simulink model "IndustrialMicrogrid"  (R2023a)
settings: Solver=FixedStepDiscrete  StartTime=0.0  StopTime=10  FixedStep=Ts  RelTol=1e-3
PostLoadFcn:
  | IndustrialMicrogridInputData
  | GfmGridFormingConverterInputParameters
model workspace (MAT data in the model file):
  caseNum = 2
undefined symbols (not defined in the file): base, BESS, DiscIntNeverNeededParam, grid, Grid, gridInverter, machine, microgrid, PV, PVInverter, PVTransformer, scrFactorRg, scrFactorXg, transformer, Ts
libraries: ee_lib x112, eeGeneralControl x104, nesl_utility_internal x64, simulink x56, nesl_utility x37, fl_lib x29, slpidlib x13, eeTransforms x11, eeTotalHarmonicDistorsion x8, eeRmsMeasurement x4, eeSinusoidalMeasurement x4, simulink_extras x2
(part 11 of 14)

== system IndustrialMicrogrid/Operator Room/OperatorControlRoom/MG1 Controller : Commands and Measurements/Microgrid Controller 1 : Commands and Measurements/Monitoring of system performance/Microgrid ==
  Frequency : Inport
  Voltage : Inport  Port=2
  Constant : Constant  Value=0
  Constant4 : Constant  Value=0
  Island Frequency MINMAX : Scope  NumInputPorts=4
  Island Voltage MINMAX : Scope  NumInputPorts=4
  MinMax Running Resettable : simulink/Math Operations/MinMax Running Resettable  Function=max  vinit=grid.frequency
  MinMax Running Resettable2 : simulink/Math Operations/MinMax Running Resettable  Function=max  vinit=1
  MinMax Running Resettable3 : simulink/Math Operations/MinMax Running Resettable  Function=min  vinit=1
  MinMax Running Resettable4 : simulink/Math Operations/MinMax Running Resettable  Function=min  vinit=grid.frequency
  Subsystem : Subsystem
  Subsystem3 : Subsystem
  start at 0.2 s1 : Subsystem
  start at 0.2 s3 : Subsystem
  wires:
  Subsystem/1(Out1) -> Island Frequency MINMAX/1  "Microgrid Frequency Croosed Low (59 HZ)"
  Constant/1 -> MinMax Running Resettable4/2, MinMax Running Resettable/2
  Frequency/1 -> start at 0.2 s3/1(In1)
  Subsystem3/1(Out1) -> Island Voltage MINMAX/1  "Microgrid Voltage Crossed Low (0.95 pu)"
  Subsystem/2(Out2) -> Island Frequency MINMAX/2  "Microgrid Frequency Crossed High (62 Hz)"
  Voltage/1 -> start at 0.2 s1/1(In1)
  MinMax Running Resettable2/1 -> Island Voltage MINMAX/3  "Microgrid Voltage Max (pu)"
  start at 0.2 s3/1(u) -> Subsystem/1(u), MinMax Running Resettable4/1, MinMax Running Resettable/1
  Subsystem3/2(Out2) -> Island Voltage MINMAX/2  "Microgrid Voltage Crossed High (1.1 pu)"
  start at 0.2 s1/1(u) -> MinMax Running Resettable3/1, MinMax Running Resettable2/1, Subsystem3/1(u)
  Constant4/1 -> MinMax Running Resettable3/2, MinMax Running Resettable2/2
  MinMax Running Resettable4/1 -> Island Frequency MINMAX/4  "Microgrid Frequency Min (Hz)"
  MinMax Running Resettable3/1 -> Island Voltage MINMAX/4  "Microgrid Voltage Min (pu)"
  MinMax Running Resettable/1 -> Island Frequency MINMAX/3  "Microgrid Frequency Max (Hz)"

== system IndustrialMicrogrid/Operator Room/OperatorControlRoom/MG1 Controller : Commands and Measurements/Microgrid Controller 1 : Commands and Measurements/Monitoring of system performance/Subsystem ==
  Active and Reactive Power : Inport
  In Bus Element1 : Inport  Port=2  PortName=mtieline1  Element=activepower
  In Bus Element6 : Inport  Port=2  PortName=mtieline1  Element=reactivepower
  In Bus Element2 : Inport  Port=3  PortName=mLoad3  Element=activepower
  In Bus Element3 : Inport  Port=3  PortName=mLoad3  Element=reactivepower
  Bus Selector : BusSelector  OutputSignals=signal1.Grid Active Power,signal1.BESS Active Power,signal1.Load Active Power,signal2.Grid Reactive Power,signal2.BESS Reactive Power,signal2.Load Reactive Power
  Constant4 : Constant  Value=0
  MinMax Running Resettable1 : simulink/Math Operations/MinMax Running Resettable  Function=max  vinit=0
  MinMax Running Resettable2 : simulink/Math Operations/MinMax Running Resettable  Function=max  vinit=0
  Sum : Sum  Inputs=++---
  Sum1 : Sum  Inputs=++---
  Terminator : Terminator
  Terminator1 : Terminator
  start at 2.5 s : Subsystem
  start at 2.5 s1 : Subsystem
  wires:
  start at 2.5 s1/1(u) -> MinMax Running Resettable2/1
  Constant4/1 -> MinMax Running Resettable1/2, MinMax Running Resettable2/2
  Sum/1 -> start at 2.5 s1/1(ActivePower)
  Sum1/1 -> start at 2.5 s/1(ReactivePower)
  Active and Reactive Power/1 -> Bus Selector/1
  MinMax Running Resettable2/1 -> Terminator/1  "Max Active Power Loss (kW)"
  start at 2.5 s/1(u) -> MinMax Running Resettable1/1
  MinMax Running Resettable1/1 -> Terminator1/1  "Max Active Power Loss (kW)"
  Bus Selector/1 -> Sum/1  "<Grid Active Power>"
  Bus Selector/2 -> Sum/2  "<BESS Active Power>"
  Bus Selector/3 -> Sum/3  "<Load Active Power>"
  Bus Selector/4 -> Sum1/1  "<Grid Reactive Power>"
  Bus Selector/5 -> Sum1/2  "<BESS Reactive Power>"
  Bus Selector/6 -> Sum1/3  "<Load Reactive Power>"
  In Bus Element1/1 -> Sum/4
  In Bus Element6/1 -> Sum1/4
  In Bus Element2/1 -> Sum/5
  In Bus Element3/1 -> Sum1/5

== system IndustrialMicrogrid/Operator Room/OperatorControlRoom/MG1 Controller : Commands and Measurements/Microgrid Controller 1 : Commands and Measurements/Monitoring of system performance/THD ==
  mLoad : Inport
  In2 : Inport  Port=2
  MGController : Inport  Port=3
  In4 : Inport  Port=4
  THD : Scope  NumInputPorts=4
  Total Harmonic Distortion{,1..3} (4 alike) : eeTotalHarmonicDistorsion/Total Harmonic Distortion  f=60  Ts=Ts
      settings: LibrarySourceBlock=|
      | ee_sl_lib/Measurements/Total Harmonic
      | Distortion
  wires:
  Total Harmonic Distortion1/1 -> THD/2  "Load Current THD (%)"
  Total Harmonic Distortion3/1 -> THD/4  "PCC Current THD (%)"
  Total Harmonic Distortion2/1 -> THD/3  "PCC Voltage THD (%)"
  Total Harmonic Distortion/1 -> THD/1  "Load Voltage THD (%)"
  In2/1 -> Total Harmonic Distortion1/1
  mLoad/1 -> Total Harmonic Distortion/1
  MGController/1 -> Total Harmonic Distortion2/1
  In4/1 -> Total Harmonic Distortion3/1

== system IndustrialMicrogrid/Operator Room/OperatorControlRoom/MG2 Controller : Commands and Measurements/Microgrid Controller 2 : Commands and Measurements/Measurements and visualizations 1/BESS, PV and Load Measurements ==
  Grid Active Power : Inport
  Grid Reactive Power : Inport  Port=2
  Vpv (V) : Inport  Port=3
  BESS Active Power : Inport  Port=4
  BESS Voltage : Inport  Port=5
  BESS Current : Inport  Port=6
  Load Active Power : Inport  Port=7
  Ipv (A) : Inport  Port=8
  PV Active Power : Inport  Port=9
  BESS Reactive Power : Inport  Port=10
  PV Reactive Power : Inport  Port=11
  Load Reactive Power : Inport  Port=12
  Load Current(p.u.) : Inport  Port=13
  Load Voltage (p.u.) : Inport  Port=14
  Load Voltage RMS (p.u.) : Inport  Port=15
  Diesel Active Power : Inport  Port=16
  Diesel Reactive Power : Inport  Port=17
  Active and reactive Power : Subsystem
  BESS and PV Measurements : Subsystem
  Load Active Power2 : InportShadow  Port=7
  Load Measurements : Subsystem
  Load Reactive Power1 : InportShadow  Port=12
  PV Active Power1 : InportShadow  Port=9
  PV Reactive Power1 : InportShadow  Port=11
  Active Power : Outport
  Reactive Power : Outport  Port=2
  wires:
  PV Reactive Power1/1 -> Active and reactive Power/8(PV Reactive Power)
  PV Active Power1/1 -> Active and reactive Power/4(PV Active Power)
  PV Active Power/1 -> BESS and PV Measurements/5(PV Active Power)
  Vpv (V)/1 -> BESS and PV Measurements/1(Vpv (V))
  PV Reactive Power/1 -> BESS and PV Measurements/6(PV Reactive Power)
  BESS Voltage/1 -> BESS and PV Measurements/2(Vabc)
  BESS Active Power/1 -> Active and reactive Power/2(BESS Active Power)
  BESS Current/1 -> BESS and PV Measurements/3(Iabc)
  Load Voltage RMS (p.u.)/1 -> Load Measurements/5(Load Voltage RMS (p.u.))
  Load Voltage (p.u.)/1 -> Load Measurements/4(Load Voltage (p.u.))
  Grid Active Power/1 -> Active and reactive Power/1(Grid Active Power)
  Load Active Power2/1 -> Load Measurements/1(Load Active Power)
  Load Reactive Power/1 -> Active and reactive Power/7(Load Reactive Power)
  Grid Reactive Power/1 -> Active and reactive Power/5(Grid Reactive Power)
  Load Active Power/1 -> Active and reactive Power/3(Load Active Power)
  Load Reactive Power1/1 -> Load Measurements/2(Load Reactive Power)
  BESS Reactive Power/1 -> Active and reactive Power/6(BESS Reactive Power)
  Load Current(p.u.)/1 -> Load Measurements/3(Load Current(p.u.))
  Ipv (A)/1 -> BESS and PV Measurements/4(Ipv (A))
  Active and reactive Power/1(Active Power) -> Active Power/1
  Active and reactive Power/2(Reactive Power) -> Reactive Power/1
  Diesel Active Power/1 -> Active and reactive Power/10(Diesel Active Power)
  Diesel Reactive Power/1 -> Active and reactive Power/9(Diesel Reactive Power)

== system IndustrialMicrogrid/Operator Room/OperatorControlRoom/MG2 Controller : Commands and Measurements/Microgrid Controller 2 : Commands and Measurements/Measurements and visualizations 1/Resynchronization and Planned Islanding ==
  Grid Frequency : Inport
  Island Frequency : Inport  Port=2
  Resynch : Inport  Port=3
  Grid Angle : Inport  Port=4
  Island Angle : Inport  Port=5
  Resynchronization : Inport  Port=6
  Grid Voltage : Inport  Port=7
  Grid Current : Inport  Port=8
  Island Voltage : Inport  Port=9
  Frequency Error : Inport  Port=10
  Grid Voltageabc1 : Inport  Port=11
  Phase Angle Error : Inport  Port=12
  Voltage Error : Inport  Port=13
  PlannedIslandCommand : Inport  Port=14
  PlannedIsland : Inport  Port=15
  Power Tracking Command : Inport  Port=16
  Grid Current1 : InportShadow  Port=8
  Grid Frequency1 : InportShadow
  Grid Voltage abc : InportShadow  Port=11
  Grid Voltage2 : InportShadow  Port=7
  Island Frequency1 : InportShadow  Port=2
  Island Voltage1 : InportShadow  Port=9
  Planned Islanding : Subsystem
  Resync : Subsystem
  wires:
  Power Tracking Command/1 -> Planned Islanding/8(Power Tracking Command)
  PlannedIsland/1 -> Planned Islanding/7(PlannedIsland)
  PlannedIslandCommand/1 -> Planned Islanding/6(PlannedIslandCommand)
  Grid Voltage2/1 -> Planned Islanding/5(Grid Voltage1)  "Grid Voltage"
  Island Voltage1/1 -> Planned Islanding/4(Island Voltage)
  Grid Current1/1 -> Planned Islanding/3(Grid Current)  "Grid Current"
  Island Frequency1/1 -> Planned Islanding/2(Island Frequency)
  Grid Frequency1/1 -> Planned Islanding/1(Grid Frequency)
  Voltage Error/1 -> Resync/13(Voltage Error)  "Voltage Error"
  Phase Angle Error/1 -> Resync/12(Phase Angle Error)  "Phase Angle Error"
  Grid Voltageabc1/1 -> Resync/11(Grid Voltage abc)  "Grid Voltage"
  Frequency Error/1 -> Resync/10(Frequency Error)  "Frequency Error"
  Island Voltage/1 -> Resync/9(Island Voltage)
  Grid Current/1 -> Resync/8(Grid Current)  "Grid Current"
  Grid Voltage/1 -> Resync/7(Grid Voltage)  "Grid Voltage"
  Resynchronization/1 -> Resync/6(Resynchronization)
  Island Angle/1 -> Resync/5(Island Angle)
  Grid Angle/1 -> Resync/4(Grid Angle)
  Resynch/1 -> Resync/3(In1)  "Resynch Command"
  Island Frequency/1 -> Resync/2(Island Frequency)
  Grid Frequency/1 -> Resync/1(Grid Frequency)
  Grid Voltage abc/1 -> Planned Islanding/9(Grid Voltage abc)  "Grid Voltage"

== system IndustrialMicrogrid/Operator Room/OperatorControlRoom/MG2 Controller : Commands and Measurements/Microgrid Controller 2 : Commands and Measurements/Monitoring of system performance/Load  ==
  In1 : Inport
  In2 : Inport  Port=2
  In3 : Inport  Port=3
  Constant1 : Constant  Value=0
  Constant2 : Constant  Value=0
  Constant3 : Constant  Value=0
  Gain : Gain  Gain=1/75
  Load Power and  Current MinMax : Scope  NumInputPorts=4
  Load Voltage MINMAX : Scope  NumInputPorts=4
  MinMax Running Resettable1 : simulink/Math Operations/MinMax Running Resettable  Function=min  vinit=1
  MinMax Running Resettable5 : simulink/Math Operations/MinMax Running Resettable  Function=max  vinit=1
  MinMax Running Resettable6 : simulink/Math Operations/MinMax Running Resettable  Function=min  vinit=0.707
  MinMax Running Resettable7 : simulink/Math Operations/MinMax Running Resettable  Function=max  vinit=0.707
  MinMax Running Resettable8 : simulink/Math Operations/MinMax Running Resettable  Function=min  vinit=0.707
  MinMax Running Resettable9 : simulink/Math Operations/MinMax Running Resettable  Function=max  vinit=0.491
  Subsystem4 : Subsystem
  start at 0.2 s2 : Subsystem
  start at 0.2 s4 : Subsystem
  start at 0.2 s5 : Subsystem
  wires:
  Constant2/1 -> MinMax Running Resettable6/2, MinMax Running Resettable7/2
  Constant1/1 -> MinMax Running Resettable1/2, MinMax Running Resettable5/2
  start at 0.2 s4/1(u) -> MinMax Running Resettable9/1, MinMax Running Resettable8/1
  MinMax Running Resettable7/1 -> Load Voltage MINMAX/4  "Load Voltage Max (pu)"
  Constant3/1 -> MinMax Running Resettable9/2, MinMax Running Resettable8/2
  MinMax Running Resettable8/1 -> Load Power and  Current MinMax/3  "Load Current Min (pu)"
  In1/1 -> start at 0.2 s2/1(In1)
  In2/1 -> start at 0.2 s4/1(In1)
  MinMax Running Resettable5/1 -> Load Power and  Current MinMax/2  "Load Power Max (pu)"
  In3/1 -> start at 0.2 s5/1(In1)
  Subsystem4/1(VoltageLow) -> Load Voltage MINMAX/1  "Load Voltage Crossed Low"
  start at 0.2 s2/1(u) -> MinMax Running Resettable7/1, MinMax Running Resettable6/1, Subsystem4/1(Voltage)
  Gain/1 -> MinMax Running Resettable5/1, MinMax Running Resettable1/1
  MinMax Running Resettable9/1 -> Load Power and  Current MinMax/4  "Load Current Max (pu)"
  start at 0.2 s5/1(u) -> Gain/1
  Subsystem4/2(VoltageHigh) -> Load Voltage MINMAX/2  "Load Voltage Crossed High"
  MinMax Running Resettable6/1 -> Load Voltage MINMAX/3  "Load Voltage Min (pu)"
  MinMax Running Resettable1/1 -> Load Power and  Current MinMax/1  "Load Power Min (pu)"

== system IndustrialMicrogrid/Operator Room/OperatorControlRoom/MG2 Controller : Commands and Measurements/Microgrid Controller 2 : Commands and Measurements/Monitoring of system performance/Microgrid ==
  Frequency : Inport
  Voltage : Inport  Port=2
  Constant : Constant  Value=0
  Constant4 : Constant  Value=0
  Island Frequency MINMAX : Scope  NumInputPorts=4
  Island Voltage MINMAX : Scope  NumInputPorts=4
  Low-Pass Filter (Discrete or Continuous) : eeGeneralControl/Low-Pass Filter (Discrete or Continuous)  K=1  T=0.04  B=inf  A=-inf  init_option=Inherited from block input  x0=0  Ts=Ts
  Low-Pass Filter (Discrete or Continuous)1 : eeGeneralControl/Low-Pass Filter (Discrete or Continuous)  K=1  T=0.04  B=inf  A=-inf  init_option=Inherited from block input  x0=0  Ts=Ts
  MinMax Running Resettable : simulink/Math Operations/MinMax Running Resettable  Function=max  vinit=grid.frequency
  MinMax Running Resettable2 : simulink/Math Operations/MinMax Running Resettable  Function=max  vinit=1
  MinMax Running Resettable3 : simulink/Math Operations/MinMax Running Resettable  Function=min  vinit=1
  MinMax Running Resettable4 : simulink/Math Operations/MinMax Running Resettable  Function=min  vinit=grid.frequency
  Subsystem : Subsystem
  Subsystem3 : Subsystem
  start at 2 s : Subsystem
  start at 2 s1 : Subsystem
  wires:
  Subsystem/1(FrequencyLow) -> Island Frequency MINMAX/1  "Microgrid Frequency Croosed Low (58.8 HZ)"
  Constant/1 -> MinMax Running Resettable4/2, MinMax Running Resettable/2
  Frequency/1 -> Low-Pass Filter (Discrete or Continuous)/1
  Subsystem3/1(VoltageLow) -> Island Voltage MINMAX/1  "Microgrid Voltage Crossed Low (0.9 pu)"
  Subsystem/2(FrequencyHigh) -> Island Frequency MINMAX/2  "Microgrid Frequency Crossed High (61.2 Hz)"
  Voltage/1 -> Low-Pass Filter (Discrete or Continuous)1/1
  MinMax Running Resettable2/1 -> Island Voltage MINMAX/3  "Microgrid Voltage Max (pu)"
  start at 2 s/1(u) -> MinMax Running Resettable4/1, MinMax Running Resettable/1, Subsystem/1(Frequency)
  Subsystem3/2(VoltageHigh) -> Island Voltage MINMAX/2  "Microgrid Voltage Crossed High (1.1 pu)"
  start at 2 s1/1(u) -> MinMax Running Resettable3/1, MinMax Running Resettable2/1, Subsystem3/1(Voltage)
  Constant4/1 -> MinMax Running Resettable3/2, MinMax Running Resettable2/2
  MinMax Running Resettable4/1 -> Island Frequency MINMAX/4  "Microgrid Frequency Min (Hz)"
  MinMax Running Resettable3/1 -> Island Voltage MINMAX/4  "Microgrid Voltage Min (pu)"
  MinMax Running Resettable/1 -> Island Frequency MINMAX/3  "Microgrid Frequency Max (Hz)"
  Low-Pass Filter (Discrete or Continuous)/1 -> start at 2 s/1(In1)
  Low-Pass Filter (Discrete or Continuous)1/1 -> start at 2 s1/1(In1)

== system IndustrialMicrogrid/Operator Room/OperatorControlRoom/MG2 Controller : Commands and Measurements/Microgrid Controller 2 : Commands and Measurements/Monitoring of system performance/Subsystem ==
  Active and Reactive Power : Inport
  In Bus Element1 : Inport  Port=2  PortName=mtieline  Element=activepower
  In Bus Element6 : Inport  Port=2  PortName=mtieline  Element=reactivepower
  Bus Selector : BusSelector  OutputSignals=signal1.Grid Active Power,signal1.Diesel Active Power,signal1.BESS Active Power,signal1.PV Active Power,signal1.Load Active Power,signal2.Grid Reactive Power,signal2.BESS Reactive Power,signal2.PV Rective Power,signal2.Diesel Reactive Power,signal2.Load Reactive Power
  Constant4 : Constant  Value=0
  MinMax Running Resettable1 : simulink/Math Operations/MinMax Running Resettable  Function=max  vinit=0
  MinMax Running Resettable2 : simulink/Math Operations/MinMax Running Resettable  Function=max  vinit=0
  Sum : Sum  Inputs=++++-+
  Sum1 : Sum  Inputs=++++-+
  Terminator : Terminator
  Terminator1 : Terminator
  start at 2.5 s : Subsystem
  start at 2.5 s1 : Subsystem
  wires:
  start at 2.5 s1/1(u) -> MinMax Running Resettable2/1
  Constant4/1 -> MinMax Running Resettable1/2, MinMax Running Resettable2/2
  Sum/1 -> start at 2.5 s1/1(ActivePower)
  Sum1/1 -> start at 2.5 s/1(ReactivePower)
  Active and Reactive Power/1 -> Bus Selector/1
  MinMax Running Resettable2/1 -> Terminator/1  "Max Active Power Loss (kW)"
  start at 2.5 s/1(u) -> MinMax Running Resettable1/1
  MinMax Running Resettable1/1 -> Terminator1/1  "Max Active Power Loss (kW)"
  Bus Selector/1 -> Sum/1  "<Grid Active Power>"
  Bus Selector/2 -> Sum/2  "<Diesel Active Power>"
  Bus Selector/3 -> Sum/3  "<BESS Active Power>"
  Bus Selector/4 -> Sum/4  "<PV Active Power>"
  Bus Selector/5 -> Sum/5  "<Load Active Power>"
  Bus Selector/6 -> Sum1/1  "<Grid Reactive Power>"
  Bus Selector/7 -> Sum1/2  "<BESS Reactive Power>"
  Bus Selector/8 -> Sum1/3  "<PV Rective Power>"
  Bus Selector/9 -> Sum1/4  "<Diesel Reactive Power>"
  Bus Selector/10 -> Sum1/5  "<Load Reactive Power>"
  In Bus Element1/1 -> Sum/6
  In Bus Element6/1 -> Sum1/6

== system IndustrialMicrogrid/Operator Room/OperatorControlRoom/MG2 Controller : Commands and Measurements/Microgrid Controller 2 : Commands and Measurements/Monitoring of system performance/THD ==
  mLoad : Inport
  In2 : Inport  Port=2
  MGController : Inport  Port=3
  In4 : Inport  Port=4
  THD : Scope  NumInputPorts=4
  Total Harmonic Distortion{,1..3} (4 alike) : eeTotalHarmonicDistorsion/Total Harmonic Distortion  f=60  Ts=Ts
  wires:
  Total Harmonic Distortion1/1 -> THD/2  "Load Current THD (%)"
  Total Harmonic Distortion3/1 -> THD/4  "PCC Current THD (%)"
  Total Harmonic Distortion2/1 -> THD/3  "PCC Voltage THD (%)"
  Total Harmonic Distortion/1 -> THD/1  "Load Voltage THD (%)"
  In2/1 -> Total Harmonic Distortion1/1
  mLoad/1 -> Total Harmonic Distortion/1
  MGController/1 -> Total Harmonic Distortion2/1
  In4/1 -> Total Harmonic Distortion3/1

== system IndustrialMicrogrid/MG1 Primary Substation/BESS and Controller/BESS/Grid-Forming Converter Control/Current Limiting/CurrentLimitingMethod/currentLimitAndVirtual ==
  Igd : Inport
  Igq : Inport  Port=2
  Current Saturation : Subsystem
  CurrentLimitSelection : Stateflow chart  TreatAsAtomicUnit=on
  Math Function : Math  Operator=hypot
  Merge{,1..3} (4 alike) : Merge  Inputs=3
  No Fault Ride Through : Subsystem
  VI : Subsystem
  delVd : Outport
  delVq : Outport  Port=2
  Idmax : Outport  Port=3
  Iqmax : Outport  Port=4
  wires:
  Merge2/1 -> Idmax/1
  Igq/1 -> Current Saturation/2(Iq), VI/2(Iq), No Fault Ride Through/2(Iq), [Iq]
  Merge1/1 -> delVq/1
  Igd/1 -> VI/1(Id), Current Saturation/1(Id), No Fault Ride Through/1(Id), [Id]
  No Fault Ride Through/1(delVd) -> Merge/3
  No Fault Ride Through/3(idmax) -> Merge2/3
  VI/1(delVd) -> Merge/1
  [Iq] -> Math Function/2
  [Id] -> Math Function/1
  Current Saturation/1(delVd) -> Merge/2
  Current Saturation/4(iqmax) -> Merge3/2
  Merge/1 -> delVd/1
  VI/2(delVq) -> Merge1/1
  Current Saturation/3(idmax) -> Merge2/2
  VI/4(iqmax) -> Merge3/1
  VI/3(idmax) -> Merge2/1
  No Fault Ride Through/4(iqmax) -> Merge3/3
  Current Saturation/2(delVq) -> Merge1/2
  Merge3/1 -> Iqmax/1
  No Fault Ride Through/2(delVq) -> Merge1/3
  Math Function/1 -> CurrentLimitSelection/1(Is)
  CurrentLimitSelection/1(ismax) -> [Imax]
  CurrentLimitSelection/2(noCurrentLimit) -> [noCtLt]
  CurrentLimitSelection/3(viCurrentLimit) -> [viCtLt]
  CurrentLimitSelection/4(satCurrentLimit) -> [satCtLt]
  [viCtLt] -> VI/Enable
  [satCtLt] -> Current Saturation/Enable
  [noCtLt] -> No Fault Ride Through/Enable
  [Imax] -> Current Saturation/3(Imaxsat)
  [Imax] -> VI/3(Imax)

== system IndustrialMicrogrid/MG1 Primary Substation/BESS and Controller/BESS/Grid-Forming Converter Control/Current Limiting/CurrentLimitingMethod/currentSaturation ==
  note: Vs-delV
  Igd : Inport
  Igq : Inport  Port=2
  Compare : Subsystem
  Constant : Constant  Value=maxSatCurrentLimit
  Constant1 : Constant  Value=0
  Constant2 : Constant  Value=0
  If : If
  If Action Subsystem : Subsystem  TreatAsAtomicUnit=on
  If Action Subsystem1 : Subsystem  TreatAsAtomicUnit=on
  Math Function : Math  Operator=hypot
  Merge : Merge
  Merge1 : Merge
  Subtract : Sum  Inputs=+-
  delVd : Outport
  delVq : Outport  Port=2
  Idmax : Outport  Port=3
  Iqmax : Outport  Port=4
  wires:
  Igd/1 -> [Isd], Math Function/1
  Igq/1 -> [Isq], Math Function/2
  Constant/1 -> Subtract/1
  Math Function/1 -> [Is], Subtract/2  "Is"
  If/1 -> If Action Subsystem/Action
  [Isd] -> If Action Subsystem/2(Isd)
  [Isq] -> If Action Subsystem/3(Isq)
  Subtract/1 -> Compare/1(u)
  Compare/1(Out1) -> If/1
  If/2 -> If Action Subsystem1/Action
  [Is] -> If Action Subsystem/1(Is)
  If Action Subsystem/1(Idmax) -> Merge/1
  If Action Subsystem1/1(Idmax) -> Merge/2
  If Action Subsystem/2(Iqmax) -> Merge1/1
  If Action Subsystem1/2(Iqmax) -> Merge1/2
  Constant2/1 -> delVq/1
  Constant1/1 -> delVd/1
  Merge/1 -> Idmax/1
  Merge1/1 -> Iqmax/1

== system IndustrialMicrogrid/MG1 Primary Substation/BESS and Controller/BESS/Grid-Forming Converter Control/Current Limiting/CurrentLimitingMethod/virtualImpedance ==
  note: X/R ratio
  note: Resistance coefficient
  Igd : Inport
  Igq : Inport  Port=2
  Constant : Constant  Value=maxVICurrentLimit
  Constant1 : Constant  Value=0
  Constant2 : Constant  Value=0
  Constant3 : Constant  Value=0
  Gain : Gain  Gain=ctLimitVirtualImp
  Gain1 : Gain  Gain=ctLimitXbyR
  Low-Pass Filter : eeGeneralControl/Low-Pass Filter (Discrete or Continuous)  K=1  T=currentVITimeConst  B=inf  A=-inf  init_option=Inherited from block input  x0=0  Ts=-1
  Math Function : Math  Operator=hypot
  Product{,1..3} (4 alike) : Product
  Relay : Relay  OnSwitchValue=0.01  OffSwitchValue=-0.05
  Saturation : Saturate  UpperLimit=1  LowerLimit=-1
  Saturation1 : Saturate  UpperLimit=1  LowerLimit=-1
  Sum : Sum  Inputs=|+-
  Sum1 : Sum  Inputs=|+-
  Sum2 : Sum  Inputs=++|
  Switch : Switch  Criteria=u2 > Threshold  SaturateOnIntegerOverflow=off  InputSameDT=off
  delVd : Outport
  delVq : Outport  Port=2
  Idmax : Outport  Port=3
  Iqmax : Outport  Port=4
  wires:
  Sum/1 -> Gain/1, Relay/1
  Igq/1 -> [Igq], Math Function/2
  Product1/1 -> Sum2/1
  Gain1/1 -> Product1/2, Product2/1
  Sum1/1 -> Saturation/1
  Product/1 -> Sum1/1
  Product2/1 -> Sum1/2
  Constant/1 -> Sum/2  "IsMaxium"
  Math Function/1 -> Low-Pass Filter/1  "Is"
  [Igq] -> Product3/1, Product2/2
  Switch/1 -> Gain1/1, Product3/2, Product/1
  [Igd] -> Product1/1, Product/2
  Constant2/1 -> Idmax/1
  Constant3/1 -> Iqmax/1
  Gain/1 -> Switch/1
  Constant1/1 -> Switch/3
  Igd/1 -> Math Function/1, [Igd]
  Saturation1/1 -> delVq/1
  Relay/1 -> Switch/2
  Saturation/1 -> delVd/1
  Low-Pass Filter/1 -> Sum/1
  Product3/1 -> Sum2/2
  Sum2/1 -> Saturation1/1

== system IndustrialMicrogrid/MG1 Primary Substation/BESS and Controller/BESS/Grid-Forming Converter Control/Grid Voltage Reactive Power Support/Modifying Active Power Reference/Computing New Active Power Ref ==
  Iq : Inport
  Vd : Inport  Port=2
  Abs : Abs  SaturateOnIntegerOverflow=off
  Constant : Constant  Value=maxVICurrentLimit*0.96
  Constant1 : Constant  Value=0
  Product : Product
  Sqrt : Sqrt
  Square : Math  Operator=square
  Square1 : Math  Operator=square
  Subtract : Sum  Inputs=-+
  Switch : Switch  Criteria=u2 > Threshold  Threshold=1.15  SaturateOnIntegerOverflow=off  InputSameDT=off
  Pref : Outport
  wires:
  Abs/1 -> Switch/3
  Constant/1 -> Square1/1
  Subtract/1 -> Sqrt/1
  Switch/1 -> Product/2
  Square/1 -> Subtract/1, Switch/2
  Square1/1 -> Subtract/2
  Constant1/1 -> Switch/1
  Vd/1 -> Product/1
  Sqrt/1 -> Abs/1
  Iq/1 -> Square/1
  Product/1 -> Pref/1

== system IndustrialMicrogrid/MG1 Primary Substation/BESS and Controller/BESS/Grid-Forming Converter Control/Grid Voltage Reactive Power Support/Modifying Reactive Power Reference/Changing the Power Reference ==
  Vs : Inport
  Vd : Inport  Port=2
  Pref : Inport  Port=3
  Qref : Inport  Port=4
  Enable : EnablePort
  ActivePowerReference : Subsystem
  Constant1 : Constant  Value=voltreference*0.96
  EstimateIdForGivenIq : Subsystem
  EstimateIqForReactivePower : Subsystem
  Max : MinMax  Function=max  Inputs=2
  ReactivePowerReference : Subsystem
  Prefv : Outport
  Qrefv : Outport  Port=2
  wires:
  EstimateIqForReactivePower/1(Iq) -> EstimateIdForGivenIq/1(Iq), ReactivePowerReference/2(Iq)
  Constant1/1 -> EstimateIqForReactivePower/1(Vmin)
  Vs/1 -> ActivePowerReference/2(Vd), EstimateIqForReactivePower/3(Vs), ReactivePowerReference/1(Vd)
  EstimateIdForGivenIq/1(Id) -> ActivePowerReference/1(Id)
  Pref/1 -> ActivePowerReference/3(Pref)
  ActivePowerReference/1(PrefNew) -> Prefv/1
  ReactivePowerReference/1(QrefNew) -> Max/1
  Max/1 -> Qrefv/1
  Qref/1 -> Max/2
  Vd/1 -> EstimateIqForReactivePower/2(Vd)

== system IndustrialMicrogrid/MG1 Primary Substation/BESS and Controller/BESS/Grid-Forming Converter Control/Grid Voltage Reactive Power Support/Modifying Reactive Power Reference/Hysteresis ==
  Vs : Inport
  AND : Logic  IconShape=distinctive  AllPortsSameDT=off  OutDataTypeStr=boolean
  Compare To Constant : simulink/Logic and Bit Operations/Compare To Constant  relop=<  const=0.9  OutDataTypeStr=boolean
  Compare To Constant1 : simulink/Logic and Bit Operations/Compare To Constant  relop=<  const=0.95  OutDataTypeStr=boolean
  D Latch : simulink_extras/Flip Flops/D Latch
  OR : Logic  Operator=OR  IconShape=distinctive  AllPortsSameDT=off  OutDataTypeStr=boolean
  Terminator : Terminator
  LVFlag : Outport
  wires:
  Compare To Constant1/1 -> AND/1
  D Latch/1 -> AND/2
  AND/1 -> OR/1
  OR/1 -> LVFlag/1
  D Latch/2 -> Terminator/1
  Compare To Constant/1 -> D Latch/1, D Latch/2, OR/2
  Vs/1 -> Compare To Constant1/1, Compare To Constant/1

== system IndustrialMicrogrid/MG1 Primary Substation/BESS and Controller/BESS/Grid-Forming Converter Control/Grid Voltage Reactive Power Support/Modifying Reactive Power Reference/Not Altering the Power Reference ==
  Pref : Inport
  Qref : Inport  Port=2
  Enable : EnablePort
  Prefv : Outport
  Qrefv : Outport  Port=2
  wires:
  Pref/1 -> Prefv/1
  Qref/1 -> Qrefv/1

== system IndustrialMicrogrid/MG1 Primary Substation/BESS and Controller/BESS/Grid-Forming Converter Control/Measurement/Frequency Measurement/Frequency Measurement ==
  abc : Inport
  Constant : Constant
  Discrete-Time Integrator : DiscreteIntegrator  SampleTime=sampleTime  LimitOutput=on  ICPrevOutput=DiscIntNeverNeededParam  ICPrevScaledInput=DiscIntNeverNeededParam
  If : If  IfExpression=u1 > 0.9
  If Action Subsystem : Subsystem  TreatAsAtomicUnit=on
  If Action Subsystem1 : Subsystem  TreatAsAtomicUnit=on
  Merge : Merge
  Postive Sequence : Subsystem
  Freq : Outport
  wires:
  If/1 -> If Action Subsystem/Action
  If/2 -> If Action Subsystem1/Action
  Discrete-Time Integrator/1 -> If Action Subsystem/2(Time), If/1
  abc/1 -> Postive Sequence/1(abc)
  Constant/1 -> Discrete-Time Integrator/1
  If Action Subsystem/1(Freq) -> Merge/1
  If Action Subsystem1/1(Out1) -> Merge/2
  Merge/1 -> Freq/1
  Postive Sequence/1(posSeq) -> If Action Subsystem/1(V)

== system IndustrialMicrogrid/MG1 Primary Substation/BESS and Controller/BESS/Grid-Forming Converter Control/Measurement/abc2dq/Supply Current to dq ==
  abc : Inport
  Angle : Inport  Port=2
  Demux : Demux  Outputs=3
  Park Transform : eeTransforms/Park Transform  AxisAlignment=D-axis  PowerInvariant=off
  Terminator : Terminator
  Igd : Outport  VectorParamsAs1DForOutWhenUnconnected=off
  Igq : Outport  Port=2  VectorParamsAs1DForOutWhenUnconnected=off
  wires:
  Demux/3 -> Terminator/1
  Park Transform/1 -> Demux/1
  Demux/2 -> Igq/1
  Demux/1 -> Igd/1
  abc/1 -> Park Transform/1
  Angle/1 -> Park Transform/2

== system IndustrialMicrogrid/MG1 Primary Substation/BESS and Controller/BESS/Grid-Forming Converter Control/Measurement/abc2dq/Supply Voltage  to dq1 ==
  Angle : Inport
  abc : Inport  Port=2
  Demux : Demux  Outputs=3
  Park Transform : eeTransforms/Park Transform  AxisAlignment=D-axis  PowerInvariant=off
  Terminator : Terminator
  Vgd : Outport  VectorParamsAs1DForOutWhenUnconnected=off
  Vgq : Outport  Port=2  VectorParamsAs1DForOutWhenUnconnected=off
  wires:
  Demux/3 -> Terminator/1
  Park Transform/1 -> Demux/1
  Demux/2 -> Vgq/1
  Demux/1 -> Vgd/1
  abc/1 -> Park Transform/1
  Angle/1 -> Park Transform/2

== system IndustrialMicrogrid/MG1 Primary Substation/BESS and Controller/BESS/Grid-Forming Converter Control/Power Control/ActivePowerControl/droopControl ==
  Pref : Inport
  Pmeas : Inport  Port=2
  fref : Inport  Port=3
  cntrlflag : Inport  Port=4
  fgrid : Inport  Port=5
  Add : Sum  Inputs=+-
  Constant : Constant
  Constant5 : Constant  Value=pi/2
  Gain : Gain  Gain=powerFreq*2*pi
  Integrator with Wrapped State (Discrete or Continuous) : eeGeneralControl/Integrator with Wrapped State (Discrete or Continuous)  LabelModeActiveChoice=Discrete  WrappedStateUpperValue=2*pi  WrappedStateLowerValue=0  x0=0  Ts=activePowerSampleTime
      settings: LibrarySourceBlock=|
      | ee_sl_lib/General Control/Integrator with
      | Wrapped State
      | (Discrete or Continuous)
  Lead-Lag (Discrete or Continuous) : eeGeneralControl/Lead-Lag (Discrete or Continuous)  T1=droopT1  T2=droopT2  B=inf  A=-inf  init_option=Inherited from block input  x0=0  Ts=activePowerSampleTime
      settings: LibrarySourceBlock=|
      | ee_sl_lib/General Control/Lead-Lag
      | (Discrete or Continuous)
  Low-Pass Filter (Discrete or Continuous) : eeGeneralControl/Low-Pass Filter (Discrete or Continuous)  K=1  T=droopTC  B=inf  A=-inf  init_option=Specify as parameter  x0=0  Ts=activePowerSampleTime
  Sum : Sum  Inputs=|-+
  Sum1 : Sum  Inputs=|-+
  Terminator : Terminator
  Terminator1 : Terminator
  Terminator2 : Terminator
  mp : Gain  Gain=droopSlope
  Theta : Outport
  w : Outport  Port=2
  wires:
  Low-Pass Filter (Discrete or Continuous)/1 -> Sum1/1
  mp/1 -> Low-Pass Filter (Discrete or Continuous)/1
  Sum/1 -> mp/1
  Pmeas/1 -> Lead-Lag (Discrete or Continuous)/1
  Add/1 -> Theta/1
  Constant5/1 -> Add/2
  Pref/1 -> Sum/1
  Gain/1 -> Integrator with Wrapped State (Discrete or Continuous)/1, w/1
  Lead-Lag (Discrete or Continuous)/1 -> Sum/2
  Integrator with Wrapped State (Discrete or Continuous)/1 -> Add/1
  Constant/1 -> Sum1/2
  Sum1/1 -> Gain/1
  fgrid/1 -> Terminator/1
  fref/1 -> Terminator1/1
  cntrlflag/1 -> Terminator2/1

== system IndustrialMicrogrid/MG1 Primary Substation/BESS and Controller/BESS/Grid-Forming Converter Control/Power Control/ActivePowerControl/vsmControl ==
  note: Measured power
  note: Damping power input
  Pref : Inport
  Pmeas : Inport  Port=2
  fref : Inport  Port=3
  cntrlflag : Inport  Port=4
  fgrid : Inport  Port=5
  Add : Sum  Inputs=+-
  Constant2 : Constant  Value=pi/2
  Damping Frequency : Subsystem  Variant=on  VariantControlMode=label  VariantControl=Choice  LabelModeActiveChoice=constFreq
  Discrete-Time Integrator : DiscreteIntegrator  IntegratorMethod=Integration: Backward Euler  InitialCondition=1  SampleTime=activePowerSampleTime  LimitOutput=on  UpperSaturationLimit=1.1  LowerSaturationLimit=0.9  ICPrevOutput=DiscIntNeverNeededParam  ICPrevScaledInput=DiscIntNeverNeededParam
  Gain : Gain  Gain=powerFreq*2*pi
  Gain1 : Gain  Gain=1/vsmInertiaTC
  Gain2 : Gain  Gain=vsmDampingConst*powerFreq
  Integrator with Wrapped State (Discrete or Continuous) : eeGeneralControl/Integrator with Wrapped State (Discrete or Continuous)  LabelModeActiveChoice=Discrete  WrappedStateUpperValue=2*pi  WrappedStateLowerValue=0  x0=0  Ts=activePowerSampleTime
      settings: LibrarySourceBlock=|
      | ee_sl_lib/General Control/Integrator with
      | Wrapped State
      | (Discrete or Continuous)
  Low-Pass Filter (Discrete or Continuous) : eeGeneralControl/Low-Pass Filter (Discrete or Continuous)  K=1  T=vsmPmeasFilterTC  B=inf  A=-inf  init_option=Specify as parameter  x0=0  Ts=activePowerSampleTime
  Power Reference Selection : Subsystem
  Saturation : Saturate  UpperLimit=dampingPowerMaxLimit  LowerLimit=dampingPowerMinLimit
  Sum1 : Sum  Inputs=-+-|
  Sum2 : Sum  Inputs=|+-
  Unit Delay : UnitDelay  SampleTime=-1  HasFrameUpgradeWarning=on
  Unit Delay1 : UnitDelay  SampleTime=-1  HasFrameUpgradeWarning=on
  Theta : Outport
  w : Outport  Port=2
  wires:
  Integrator with Wrapped State (Discrete or Continuous)/1 -> Add/1
  Sum1/1 -> Gain1/1  "Pinertia"
  Constant2/1 -> Add/2
  Add/1 -> Theta/1
  Discrete-Time Integrator/1 -> Gain/1, Unit Delay1/1, Sum2/1
  Low-Pass Filter (Discrete or Continuous)/1 -> Sum1/1
  Gain2/1 -> Saturation/1
  Power Reference Selection/1(power) -> Sum1/2
  Sum2/1 -> Unit Delay/1
  Gain1/1 -> Discrete-Time Integrator/1
  Gain/1 -> Integrator with Wrapped State (Discrete or Continuous)/1, w/1
  Unit Delay/1 -> Gain2/1
  Unit Delay1/1 -> [Wsm]
  Saturation/1 -> Sum1/3  "Pdamping"
  fgrid/1 -> Damping Frequency/1(fref)
  Damping Frequency/1(fmeas) -> Sum2/2
  cntrlflag/1 -> Power Reference Selection/1(cntrlflag)
  Pref/1 -> Power Reference Selection/2(Pref)
  fref/1 -> Power Reference Selection/3(fref)
  Pmeas/1 -> Low-Pass Filter (Discrete or Continuous)/1
  [Wsm] -> Power Reference Selection/4(Wsm)

== system IndustrialMicrogrid/MG1 Primary Substation/BESS and Controller/BESS/Grid-Forming Converter Control/Power Control/ReactiveControl/Voltage  Reference Selection ==
  cntrlflag : Inport
  Qref : Inport  Port=2
  Qmeas : Inport  Port=3
  Vref : Inport  Port=4
  Vgdmeas : Inport  Port=5
  If : If
  If Action Subsystem : Subsystem  TreatAsAtomicUnit=on
  If Action Subsystem1 : Subsystem  TreatAsAtomicUnit=on
  Merge : Merge
  Rate Transition : RateTransition
  Vd : Outport
  wires:
  If/1 -> If Action Subsystem/Action
  If Action Subsystem/1(Vd) -> Merge/1
  If/2 -> If Action Subsystem1/Action
  cntrlflag/1 -> Rate Transition/1
  Merge/1 -> Vd/1
  Qmeas/1 -> If Action Subsystem/2(Qmeas)
  Qref/1 -> If Action Subsystem/1(Qref)
  If Action Subsystem1/1(Voltage) -> Merge/2
  Vref/1 -> If Action Subsystem1/1(Vref)
  Vgdmeas/1 -> If Action Subsystem1/2(Vmeas)
  Rate Transition/1 -> If/1

== system IndustrialMicrogrid/MG1 Primary Substation/BESS and Controller/BESS/Grid-Forming Converter Control/VoltageCurrentControl/Controller/Id Current Limiting ==
  Imax : Inport
  Id : Inport  Port=2
  Abs : Abs  SaturateOnIntegerOverflow=off
  Switch : Switch  Criteria=u2 > Threshold  SaturateOnIntegerOverflow=off  InputSameDT=off
  Idref : Outport
  wires:
  Id/1 -> Switch/3
  Abs/1 -> Switch/2
  Imax/1 -> Abs/1, Switch/1
  Switch/1 -> Idref/1

== system IndustrialMicrogrid/MG1 Primary Substation/BESS and Controller/BESS/Grid-Forming Converter Control/VoltageCurrentControl/Controller/Iq Current Limiting ==
  Imax : Inport
  Iq : Inport  Port=2
  Abs : Abs  SaturateOnIntegerOverflow=off
  Switch : Switch  Criteria=u2 > Threshold  SaturateOnIntegerOverflow=off  InputSameDT=off
  Iqref : Outport
  wires:
  Iq/1 -> Switch/3
  Abs/1 -> Switch/2
  Imax/1 -> Abs/1, Switch/1
  Switch/1 -> Iqref/1

== system IndustrialMicrogrid/MG1 Primary Substation/BESS and Controller/BESS/Grid-Forming Converter Control/VoltageCurrentControl/Controller/Voltage control ==
  e : Inport
  resetBlackStart : Inport  Port=2
  Discrete-Time Integrator : DiscreteIntegrator  IntegratorMethod=Integration: Backward Euler  ExternalReset=level  SampleTime=voltControlTs  LimitOutput=on  UpperSaturationLimit=VdMaxCt  LowerSaturationLimit=VdMinCt  ICPrevOutput=DiscIntNeverNeededParam  ICPrevScaledInput=DiscIntNeverNeededParam
  Ki : Gain  Gain=VdIGain
  Kp : Gain  Gain=vdPGain
  Limit : Saturate  UpperLimit=VdMaxCt  LowerLimit=VdMinCt
  Sum7 : Sum  Inputs=|++
  u : Outport  VectorParamsAs1DForOutWhenUnconnected=off
  wires:
  Discrete-Time Integrator/1 -> Sum7/2
  Kp/1 -> Sum7/1
  Limit/1 -> u/1
  Ki/1 -> Discrete-Time Integrator/1
  Sum7/1 -> Limit/1
  e/1 -> Kp/1, Ki/1
  resetBlackStart/1 -> Discrete-Time Integrator/2

== system IndustrialMicrogrid/MG1 Primary Substation/BESS and Controller/BESS/Grid-Forming Converter Control/VoltageCurrentControl/Controller/Voltage control1 ==
  e : Inport
  resetBlackStart : Inport  Port=2
  Discrete-Time Integrator : DiscreteIntegrator  IntegratorMethod=Integration: Backward Euler  ExternalReset=level  SampleTime=voltControlTs  LimitOutput=on  UpperSaturationLimit=VqMaxCt  LowerSaturationLimit=VqMinCt  ICPrevOutput=DiscIntNeverNeededParam  ICPrevScaledInput=DiscIntNeverNeededParam
  Ki : Gain  Gain=VqIGain
  Kp : Gain  Gain=VqPGain
  Limit : Saturate  UpperLimit=VqMaxCt  LowerLimit=VqMinCt
  Sum7 : Sum  Inputs=|++
  u : Outport  VectorParamsAs1DForOutWhenUnconnected=off
  wires:
  Discrete-Time Integrator/1 -> Sum7/2
  Sum7/1 -> Limit/1
  e/1 -> Ki/1, Kp/1
  Kp/1 -> Sum7/1
  Ki/1 -> Discrete-Time Integrator/1
  Limit/1 -> u/1
  resetBlackStart/1 -> Discrete-Time Integrator/2

== system IndustrialMicrogrid/MG1 Primary Substation/BESS and Controller/BESS/Grid-Forming Converter Control/VoltageCurrentControl/Controller/d-axis current control ==
  e : Inport
  resetBlackStart : Inport  Port=2
  Discrete-Time Integrator : DiscreteIntegrator  IntegratorMethod=Integration: Backward Euler  ExternalReset=level  SampleTime=currentControlTs  LimitOutput=on  UpperSaturationLimit=4  LowerSaturationLimit=-4  ICPrevOutput=DiscIntNeverNeededParam  ICPrevScaledInput=DiscIntNeverNeededParam
  Ki : Gain  Gain=IdIGain
  Kp : Gain  Gain=IdPGain
  Limit : Saturate  UpperLimit=4  LowerLimit=-4
  Sum7 : Sum  Inputs=|++
  u : Outport  VectorParamsAs1DForOutWhenUnconnected=off
  wires:
  Discrete-Time Integrator/1 -> Sum7/2
  Sum7/1 -> Limit/1
  e/1 -> Ki/1, Kp/1
  Kp/1 -> Sum7/1
  Limit/1 -> u/1
  Ki/1 -> Discrete-Time Integrator/1
  resetBlackStart/1 -> Discrete-Time Integrator/2

== system IndustrialMicrogrid/MG1 Primary Substation/BESS and Controller/BESS/Grid-Forming Converter Control/VoltageCurrentControl/Controller/q-axis current control ==
  e : Inport
  resetBlackStart : Inport  Port=2
  Discrete-Time Integrator : DiscreteIntegrator  IntegratorMethod=Integration: Backward Euler  ExternalReset=level  SampleTime=currentControlTs  LimitOutput=on  UpperSaturationLimit=3  LowerSaturationLimit=-3  ICPrevOutput=DiscIntNeverNeededParam  ICPrevScaledInput=DiscIntNeverNeededParam
  Ki : Gain  Gain=IqIGain
  Kp : Gain  Gain=IqPGain
  Limit : Saturate  UpperLimit=3  LowerLimit=-3
  Sum7 : Sum  Inputs=|++
  u : Outport  VectorParamsAs1DForOutWhenUnconnected=off
  wires:
  Ki/1 -> Discrete-Time Integrator/1
  Kp/1 -> Sum7/1
  e/1 -> Kp/1, Ki/1
  Sum7/1 -> Limit/1
  Limit/1 -> u/1
  Discrete-Time Integrator/1 -> Sum7/2
  resetBlackStart/1 -> Discrete-Time Integrator/2

== system IndustrialMicrogrid/MG2 PV Plant/(500KWp PV)/PV Inverter A2/PV Controller/DC voltage controller & current reference/Subsystem1/V_dc_Controller1 ==
  PV_plant1 : Inport
  In2 : Inport  Port=2
  Gain : Gain  Gain=1/PV.controllerVdcBase
  PID Controller : slpidlib/PID Controller  Controller=PID  Form=Ideal  TimeDomain=Discrete-time  UseExternalTs=off  SampleTime=-1  IntegratorMethod=Forward Euler  FilterMethod=Forward Euler  ControllerParametersSource=internal  P=PV.controllerKpv*0.01  I=PV.controllerKiv*0.1  UseKiTs=off  D=PV.controllerKdv  N=100  UseFilter=on  TunerSelectOption=Transfer Function Based (PID Tuner App)  ZeroCross=off  InitialConditionSource=internal  InitialConditionForIntegrator=2.5e-7  InitialConditionForFilter=0  DifferentiatorICPrevScaledInput=0  ExternalReset=none  TrackingMode=off  Kt=1  LimitOutput=off  SatLimitsSource=internal  UpperSaturationLimit=inf  LowerSaturationLimit=-inf  LinearizeAsGain=on  AntiWindupMode=none  Kb=1  LimitIntegrator=off  UpperIntegratorSaturationLimit=inf  LowerIntegratorSaturationLimit=-inf  POutMin=[]  POutMax=[]  IOutMin=[]  IOutMax=[]  DOutMin=[]  DOutMax=[]  NOutMin=[]  NOutMax=[]  SumOutMin=[]  SumOutMax=[]  SaturationOutMin=[]  SaturationOutMax=[]  PParamMin=[]  PParamMax=[]  IParamMin=[]  IParamMax=[]  DParamMin=[]  DParamMax=[]  NParamMin=[]  NParamMax=[]  KbParamMin=[]  KbParamMax=[]  KtParamMin=[]  KtParamMax=[]  KbOutMin=[]  KbOutMax=[]  KtOutMin=[]  KtOutMax=[]  IntegratorOutMin=[]  IntegratorOutMax=[]  FilterOutMin=[]  FilterOutMax=[]  SumI1OutMin=[]  SumI1OutMax=[]  SumI2OutMin=[]  SumI2OutMax=[]  SumI3OutMin=[]  SumI3OutMax=[]  SumI4OutMin=[]  SumI4OutMax=[]  SumDOutMin=[]  SumDOutMax=[]  DifferentiatorOutMin=[]  DifferentiatorOutMax=[]  FilterDiffOutCoefMin=[]  FilterDiffOutCoefMax=[]  ReciprocalOutMin=[]  ReciprocalOutMax=[]  SumDenOutMin=[]  SumDenOutMax=[]  SumNumOutMin=[]  SumNumOutMax=[]  DivideOutMin=[]  DivideOutMax=[]  UdiffTsProdOutMin=[]  UdiffTsProdOutMax=[]  NTsProdOutMin=[]  NTsProdOutMax=[]  UintegralTsProdOutMin=[]  UintegralTsProdOutMax=[]  UngainTsProdOutMin=[]  UngainTsProdOutMax=[]  ClampingZeroOutDataTypeStr=Inherit: Inherit via back propagation  ClampingZeroOutMin=[]  ClampingZeroOutMax=[]  FilterDenConstantOutDataTypeStr=Inherit: Inherit via back propagation  FilterDenConstantOutMin=[]  FilterDenConstantOutMax=[]  PCopyOutDataTypeStr=Inherit: Inherit via back propagation  PCopyOutMin=[]  PCopyOutMax=[]  NCopyOutDataTypeStr=Inherit: Inherit via back propagation  NCopyOutMin=[]  NCopyOutMax=[]  IntegratorContinuousStateAttributes=''  IntegratorStateMustResolveToSignalObject=off  IntegratorRTWStateStorageClass=Auto  FilterContinuousStateAttributes=''  FilterStateMustResolveToSignalObject=off  FilterRTWStateStorageClass=Auto  ParallelPVariant=Passthrough  IdealPVariant=InternalParameters  IVariant=InternalParameters  DVariant=InternalParameters  IntegratorVariant=Discrete  SatVariant=Disabled  AWVariant=Passthrough  PCopyVariant=Disabled  TRVariant=Disabled  FdbkBlocksVariant=Forward  IdealPFdbkVariant=Disabled  SatFdbkVariant=Disabled  DerivativeFilterVariant=ForwardEulerFilter  NVariant=InternalParameters  NCopyVariant=Disabled  FilterICVariant=InternalICsFilter  IntegratorICVariant=InternalICs  ExternalResetVariant=Disabled  TRSumVariant=Passthrough  SumFdbkVariant=Disabled  SumVariant=Sum_PID  TsampFilterVariant=InternalTs  TsampNgainVariant=Passthrough  TsampIntegralVariant=Disabled_SignalSpec  ExternalSaturationOutDataTypeStr=Inherit: Same as second input
  Sum : Sum  Inputs=|+-
  Out1 : Outport
  wires:
  Sum/1 -> Gain/1
  Gain/1 -> PID Controller/1
  PID Controller/1 -> Out1/1
  In2/1 -> Sum/2
  PV_plant1/1 -> Sum/1

== system IndustrialMicrogrid/MG2 Primary Substation/BESS and Controller 2/BESS/Grid-Forming Converter Control/Current Limiting/CurrentLimitingMethod/currentLimitAndVirtual ==
  Igd : Inport
  Igq : Inport  Port=2
  Current Saturation : Subsystem
  CurrentLimitSelection : Stateflow chart  TreatAsAtomicUnit=on
  Math Function : Math  Operator=hypot
  Merge{,1..3} (4 alike) : Merge  Inputs=3
  No Fault Ride Through : Subsystem
  VI : Subsystem
  delVd : Outport
  delVq : Outport  Port=2
  Idmax : Outport  Port=3
  Iqmax : Outport  Port=4
  wires:
  Merge2/1 -> Idmax/1
  Igq/1 -> Current Saturation/2(Iq), VI/2(Iq), No Fault Ride Through/2(Iq), [Iq]
  Merge1/1 -> delVq/1
  Igd/1 -> VI/1(Id), Current Saturation/1(Id), No Fault Ride Through/1(Id), [Id]
  No Fault Ride Through/1(delVd) -> Merge/3
  No Fault Ride Through/3(idmax) -> Merge2/3
  VI/1(delVd) -> Merge/1
  [Iq] -> Math Function/2
  [Id] -> Math Function/1
  Current Saturation/1(delVd) -> Merge/2
  Current Saturation/4(iqmax) -> Merge3/2
  Merge/1 -> delVd/1
  VI/2(delVq) -> Merge1/1
  Current Saturation/3(idmax) -> Merge2/2
  VI/4(iqmax) -> Merge3/1
  VI/3(idmax) -> Merge2/1
  No Fault Ride Through/4(iqmax) -> Merge3/3
  Current Saturation/2(delVq) -> Merge1/2
  Merge3/1 -> Iqmax/1
  No Fault Ride Through/2(delVq) -> Merge1/3
  Math Function/1 -> CurrentLimitSelection/1(Is)
  CurrentLimitSelection/1(ismax) -> [Imax]
  CurrentLimitSelection/2(noCurrentLimit) -> [noCtLt]
  CurrentLimitSelection/3(viCurrentLimit) -> [viCtLt]
  CurrentLimitSelection/4(satCurrentLimit) -> [satCtLt]
  [viCtLt] -> VI/Enable
  [satCtLt] -> Current Saturation/Enable
  [noCtLt] -> No Fault Ride Through/Enable
  [Imax] -> Current Saturation/3(Imaxsat)
  [Imax] -> VI/3(Imax)

== system IndustrialMicrogrid/MG2 Primary Substation/BESS and Controller 2/BESS/Grid-Forming Converter Control/Current Limiting/CurrentLimitingMethod/currentSaturation ==
  note: Vs-delV
  Igd : Inport
  Igq : Inport  Port=2
  Compare : Subsystem
  Constant : Constant  Value=maxSatCurrentLimit
  Constant1 : Constant  Value=0
  Constant2 : Constant  Value=0
  If : If
  If Action Subsystem : Subsystem  TreatAsAtomicUnit=on
  If Action Subsystem1 : Subsystem  TreatAsAtomicUnit=on
  Math Function : Math  Operator=hypot
  Merge : Merge
  Merge1 : Merge
  Subtract : Sum  Inputs=+-
  delVd : Outport
  delVq : Outport  Port=2
  Idmax : Outport  Port=3
  Iqmax : Outport  Port=4
  wires:
  Igd/1 -> [Isd], Math Function/1
  Igq/1 -> [Isq], Math Function/2
  Constant/1 -> Subtract/1
  Math Function/1 -> [Is], Subtract/2  "Is"
  If/1 -> If Action Subsystem/Action
  [Isd] -> If Action Subsystem/2(Isd)
  [Isq] -> If Action Subsystem/3(Isq)
  Subtract/1 -> Compare/1(u)
  Compare/1(Out1) -> If/1
  If/2 -> If Action Subsystem1/Action
  [Is] -> If Action Subsystem/1(Is)
  If Action Subsystem/1(Idmax) -> Merge/1
  If Action Subsystem1/1(Idmax) -> Merge/2
  If Action Subsystem/2(Iqmax) -> Merge1/1
  If Action Subsystem1/2(Iqmax) -> Merge1/2
  Constant2/1 -> delVq/1
  Constant1/1 -> delVd/1
  Merge/1 -> Idmax/1
  Merge1/1 -> Iqmax/1

== system IndustrialMicrogrid/MG2 Primary Substation/BESS and Controller 2/BESS/Grid-Forming Converter Control/Current Limiting/CurrentLimitingMethod/virtualImpedance ==
  note: X/R ratio
  note: Resistance coefficient
  Igd : Inport
  Igq : Inport  Port=2
  Constant : Constant  Value=maxVICurrentLimit
  Constant1 : Constant  Value=0
  Constant2 : Constant  Value=0
  Constant3 : Constant  Value=0
  Gain : Gain  Gain=ctLimitVirtualImp
  Gain1 : Gain  Gain=ctLimitXbyR
  Low-Pass Filter : eeGeneralControl/Low-Pass Filter (Discrete or Continuous)  K=1  T=currentVITimeConst  B=inf  A=-inf  init_option=Inherited from block input  x0=0  Ts=-1
  Math Function : Math  Operator=hypot
  Product{,1..3} (4 alike) : Product
  Relay : Relay  OnSwitchValue=0.01  OffSwitchValue=-0.05
  Saturation : Saturate  UpperLimit=1  LowerLimit=-1
  Saturation1 : Saturate  UpperLimit=1  LowerLimit=-1
  Sum : Sum  Inputs=|+-
  Sum1 : Sum  Inputs=|+-
  Sum2 : Sum  Inputs=++|
  Switch : Switch  Criteria=u2 > Threshold  SaturateOnIntegerOverflow=off  InputSameDT=off
  delVd : Outport
  delVq : Outport  Port=2
  Idmax : Outport  Port=3
  Iqmax : Outport  Port=4
  wires:
  Sum/1 -> Gain/1, Relay/1
  Igq/1 -> [Igq], Math Function/2
  Product1/1 -> Sum2/1
  Gain1/1 -> Product1/2, Product2/1
  Sum1/1 -> Saturation/1
  Product/1 -> Sum1/1
  Product2/1 -> Sum1/2
  Constant/1 -> Sum/2  "IsMaxium"
  Math Function/1 -> Low-Pass Filter/1  "Is"
  [Igq] -> Product3/1, Product2/2
  Switch/1 -> Gain1/1, Product3/2, Product/1
  [Igd] -> Product1/1, Product/2
  Constant2/1 -> Idmax/1
  Constant3/1 -> Iqmax/1
  Gain/1 -> Switch/1
  Constant1/1 -> Switch/3
  Igd/1 -> Math Function/1, [Igd]
  Saturation1/1 -> delVq/1
  Relay/1 -> Switch/2
  Saturation/1 -> delVd/1
  Low-Pass Filter/1 -> Sum/1
  Product3/1 -> Sum2/2
  Sum2/1 -> Saturation1/1

== system IndustrialMicrogrid/MG2 Primary Substation/BESS and Controller 2/BESS/Grid-Forming Converter Control/Grid Voltage Reactive Power Support/Modifying Active Power Reference/Computing New Active Power Ref ==
  Iq : Inport
  Vd : Inport  Port=2
  Abs : Abs  SaturateOnIntegerOverflow=off
  Constant : Constant  Value=maxVICurrentLimit*0.96
  Constant1 : Constant  Value=0
  Product : Product
  Sqrt : Sqrt
  Square : Math  Operator=square
  Square1 : Math  Operator=square
  Subtract : Sum  Inputs=-+
  Switch : Switch  Criteria=u2 > Threshold  Threshold=1.15  SaturateOnIntegerOverflow=off  InputSameDT=off
  Pref : Outport
  wires:
  Abs/1 -> Switch/3
  Constant/1 -> Square1/1
  Subtract/1 -> Sqrt/1
  Switch/1 -> Product/2
  Square/1 -> Subtract/1, Switch/2
  Square1/1 -> Subtract/2
  Constant1/1 -> Switch/1
  Vd/1 -> Product/1
  Sqrt/1 -> Abs/1
  Iq/1 -> Square/1
  Product/1 -> Pref/1
